simulink model "my_system_ml"  (R2023a)
settings: Solver=VariableStepAuto  StartTime=0.0  StopTime=0.5  MaxStep=1e-6  RelTol=1e-3
undefined symbols (not defined in the file or in its folder): DiscIntNeverNeededParam, Ts, Ts_motor
libraries: slpidlib x50, nesl_utility x20, ee_lib x10, fl_lib x9, simulink x2, rllib x2, spsPWMGeneratorDCDCLib x1, sdl_lib x1, aerolibatmos2 x1
(part 1 of 2)
settings Model: Creator=evloev.saifuddin  LastModifiedBy=evloev.saifuddin

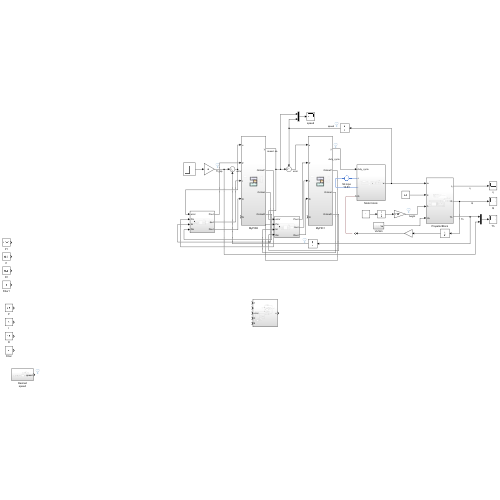
[thumbnail: Simulink's stored preview of the top-level diagram]
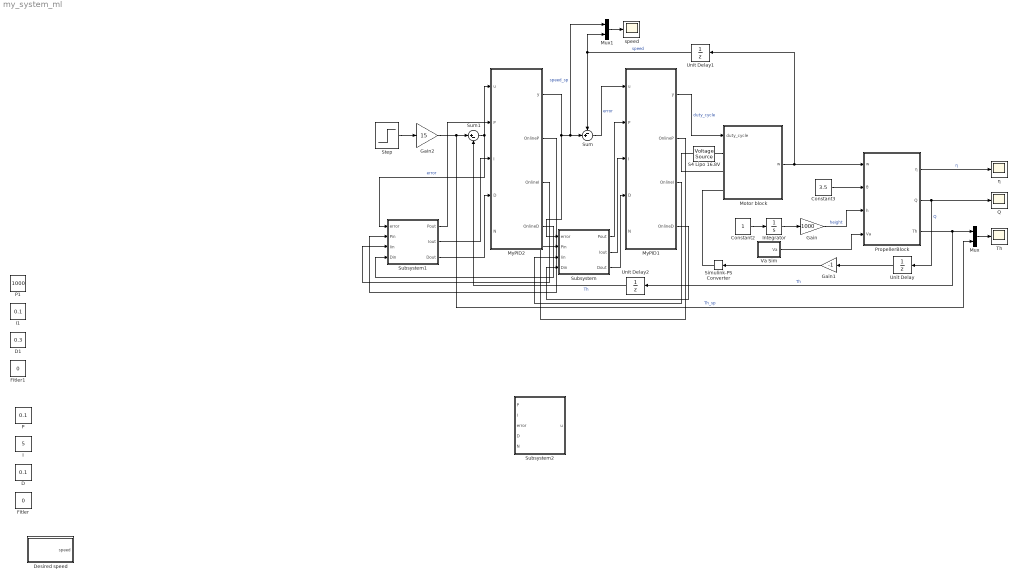
== system my_system_ml ==
  Constant2 : Constant
  Constant3 : Constant  Value=3.5
  D : Constant  Value=0.1
  D1 : Constant  Value=0.3
  Desired speed : Subsystem
  Fitler : Constant  Value=0
  Fitler1 : Constant  Value=0
  Gain : Gain  Gain=1000
  Gain1 : Gain  Gain=-1
  Gain2 : Gain  Gain=15
  I : Constant  Value=5
  I1 : Constant  Value=0.1
  Integrator : Integrator
  Motor block : Subsystem
  Mux : Mux  Inputs=2
  Mux1 : Mux  Inputs=2
  MyPID1 : Subsystem
  MyPID2 : Subsystem
  P : Constant  Value=0.1
  P1 : Constant  Value=1000
  PropellerBlock : Subsystem
  Q : Scope
  S4 Lipo 16.8V : ee_lib/Sources/Voltage Source  dc_voltage=500 V  ac_voltage=0 V  ac_shift=0 rad  ac_frequency=0 Hz  noise_mode=ee.enum.sources.noise.Disabled  PSD=0 V^2/Hz  sample_time=1e-3 s  repeatability=ee.enum.sources.repeatability.NotRepeatable  user_seed=0  auto_seed=19903842  i_specify=off  i_priority=None  i=0 A  i_nominal_specify=off  i_nominal_unit=A  i_nominal_value=1  v_specify=off  v_priority=None  v=0 V  v_nominal_specify=off  v_nominal_unit=V  v_nominal_value=1
  Simulink-PS Converter : nesl_utility/Simulink-PS Converter  PhysicalDomain=network_engine_domain  SubClassName=ps_input  LeftPortType=input  RightPortType=output  PseudoPeriodic=off  Frequencies=[]  NoiseDistribution=none  NoiseParameters=[]  Unit=N*m  AffineConversion=off  FilteringAndDerivatives=provide  SimscapeFilterOrder=1  InputFilterTimeConstant=0.001  UdotUserProvided=0
  Step : Step  Time=0.1  SampleTime=0
  Subsystem : Subsystem
  Subsystem1 : Subsystem
  Subsystem2 : Subsystem
  Sum : Sum  Inputs=-+|
  Sum1 : Sum  Inputs=|+-
  Th : Scope
  Unit Delay : UnitDelay  SampleTime=-1  HasFrameUpgradeWarning=on
  Unit Delay1 : UnitDelay  SampleTime=-1  HasFrameUpgradeWarning=on
  Unit Delay2 : UnitDelay  SampleTime=-1  HasFrameUpgradeWarning=on
  Va Sim : Subsystem
  speed : Scope
  η : Scope
  wires:
  Integrator/1 -> Gain/1
  PropellerBlock/1(η) -> η/1  "η"
  Constant3/1 -> PropellerBlock/2(θ)
  PropellerBlock/3(Th) -> Mux/1, Unit Delay2/1  "Th"
  Gain/1 -> PropellerBlock/3(h)  "height"
  Constant2/1 -> Integrator/1
  Unit Delay/1 -> Gain1/1
  PropellerBlock/2(Q) -> Unit Delay/1, Q/1  "Q"
  Gain1/1 -> Simulink-PS Converter/1
  Unit Delay1/1 -> Mux1/2, Sum/1  "speed"
  Va Sim/1(Va) -> PropellerBlock/4(Va)
  MyPID2/1(y) -> Subsystem/1(error), Mux1/1, Sum/2  "speed_sp"
  Sum1/1 -> MyPID2/1(u), Subsystem1/1(error)  "error"
  Gain2/1 -> Mux/2, Sum1/1  "Th_sp"
  Unit Delay2/1 -> Sum1/2  "Th"
  Motor block/1(w) -> Unit Delay1/1, PropellerBlock/1(w)
  Sum/1 -> MyPID1/1(u)  "error"
  MyPID1/1(y) -> Motor block/1(duty_cycle)  "duty_cycle"
  Mux/1 -> Th/1
  Step/1 -> Gain2/1
  Mux1/1 -> speed/1
  MyPID1/2(OnlineP) -> Subsystem/2(Pin)
  MyPID1/3(OnlineI) -> Subsystem/3(Iin)
  MyPID1/4(OnlineD) -> Subsystem/4(Din)
  Subsystem/1(Pout) -> MyPID1/2(P)
  Subsystem/2(Iout) -> MyPID1/3(I)
  Subsystem/3(Dout) -> MyPID1/4(D)
  Subsystem1/1(Pout) -> MyPID2/2(P)
  Subsystem1/2(Iout) -> MyPID2/3(I)
  Subsystem1/3(Dout) -> MyPID2/4(D)
  MyPID2/4(OnlineD) -> Subsystem1/4(Din)
  MyPID2/3(OnlineI) -> Subsystem1/3(Iin)
  MyPID2/2(OnlineP) -> Subsystem1/2(Pin)
  connections:
  S4 Lipo 16.8V/LConn1 -- Motor block/LConn1
  S4 Lipo 16.8V/RConn1 -- Motor block/LConn2
  Simulink-PS Converter/RConn1 -- Motor block/LConn3

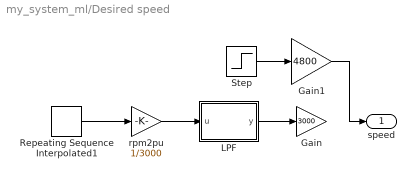
== system my_system_ml/Desired speed ==
  Gain : Gain  Gain=3000
  Gain1 : Gain  Gain=4800
  LPF : Subsystem
  Repeating Sequence Interpolated1 : simulink/Sources/Repeating Sequence Interpolated  OutValues=[0 1025/2 1025/2 1025 1025 2050 2050 2050]  TimeValues=[0 1 2 3 4 5 6 7]/2  LookUpMeth=Interpolation-Use End Values  tsamp=Ts_motor  OutMin=[]  OutMax=[]  OutDataTypeStr=double  OutputDataTypeScalingMode=double  OutDataType=fixdt(0,8)  OutScaling=2^-10
  Step : Step  Time=0.1  SampleTime=0
  rpm2pu : Gain  Gain=1/3000  RndMeth=Simplest  OutDataTypeStr=Inherit: Same as input
  speed : Outport
  wires:
  Repeating Sequence Interpolated1/1 -> rpm2pu/1
  rpm2pu/1 -> LPF/1(u)
  LPF/1(y) -> Gain/1
  Step/1 -> Gain1/1
  Gain1/1 -> speed/1

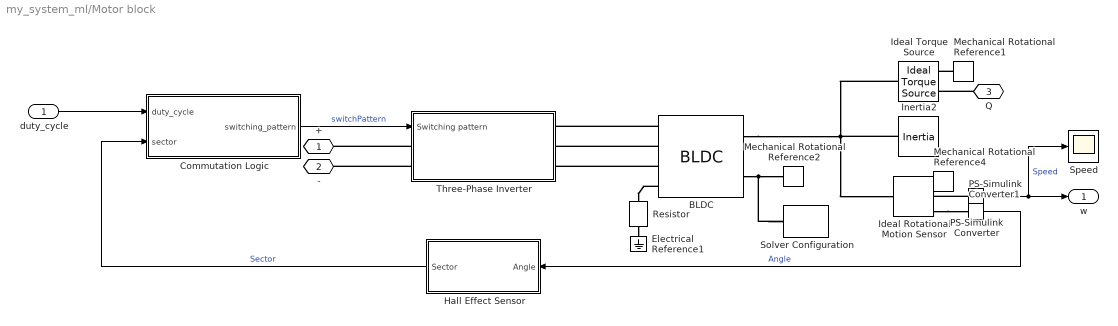
== system my_system_ml/Motor block ==
  duty_cycle : Inport
  BLDC : ee_lib/Electromechanical/Permanent Magnet/BLDC  port_option=ee.enum.threePhasePort.expanded  winding_type=ee.enum.statorconnection.wye  rotor_param=1  pm_flux_linkage=0.00043 Wb  theta_constant=120/7 deg  emf_max=9.6 V  w_meas=600 rpm  DphiDtheta_tab=[0, -.1528, -.1528, .1528, .1528, 0] Wb/rad  back_emf_tab=[0, -9.6, -9.6, 9.6, 9.6, 0] V  rotor_angle_tab=[0, 7.5, 22.5, 37.5, 52.5, 60] deg  nPolePairs=7  axes_param=ee.enum.rotorangle.qaxis  stator_param=ee.enum.statorparam.LdLqL0  machine_param=ee.enum.dqparameterization.constant  Ld=0.000022 H  Lq=0.000022 H  idVec=[-200, 0, 200] A  iqVec=[-200, 0, 200] A  LdMatrix=0.00022 * ones(3, 3) H  LqMatrix=0.00022 * ones(3, 3) H  L0=0.00016 H  Ls=0.0002 H  Lm=0 H  Ms=0.00002 H  Rs=37 mOhm  zero_sequence=ee.enum.park.zerosequence.include  loss_param=ee.enum.ironloss.none  losses_oc=[0, 0, 0] W  losses_sc=[0, 0, 0] W  f_losses=60 Hz  Isc_losses=95 A  J=1.5e-6 kg*m^2  lam=1e-7 N*m/(rad/s)  i_d_specify=off  i_d_priority=None  i_d=0 A  i_d_nominal_specify=off  i_d_nominal_unit=A  i_d_nominal_value=1  i_q_specify=off  i_q_priority=None  i_q=0 A  i_q_nominal_specify=off  i_q_nominal_unit=A  i_q_nominal_value=1  torque_specify=off  torque_priority=None  torque=0 N*m  torque_nominal_specify=off  torque_nominal_unit=N*m  torque_nominal_value=1  angular_velocity_specify=off  angular_velocity_priority=High  angular_velocity=0 rpm  angular_velocity_nominal_specify=off  angular_velocity_nominal_unit=rpm  angular_velocity_nominal_value=1  angular_position_specify=off  angular_position_priority=High  angular_position=0 deg  angular_position_nominal_specify=off  angular_position_nominal_unit=deg  angular_position_nominal_value=1  alpha=3.93e-3 1/K  alpha_flux=-0.001 1/K  Tmeas=298.15 K  stator_thermal_mass=100 J/K  rotor_thermal_mass=200 J/K  Rm_percent_rotor=90  Rd_percent_rotor=30  temperatureA_specify=off  temperatureA_priority=High  temperatureA=25 degC  temperatureA_nominal_specify=off  temperatureA_nominal_unit=degC  temperatureA_nominal_value=1  temperatureB_specify=off  temperatureB_priority=High  temperatureB=25 degC  temperatureB_nominal_specify=off  temperatureB_nominal_unit=degC  temperatureB_nominal_value=1  temperatureC_specify=off  temperatureC_priority=High  temperatureC=25 degC  temperatureC_nominal_specify=off  temperatureC_nominal_unit=degC  temperatureC_nominal_value=1  temperatureR_specify=off  temperatureR_priority=High  temperatureR=25 degC  temperatureR_nominal_specify=off  temperatureR_nominal_unit=degC  temperatureR_nominal_value=1
      settings: InternalSimscapePortConfiguration="{\"Bottom\":[],\"Left\":[{\"id\":\"a\",\"label\":\"a\",\"type\":\"foundation.electrical.electrical\"},{\"id\":\"b\",\"label\":\"b\",\"type\":\"foundation.electrical.electrical\"},{\"id\":\"c\",\"label\":\"c\",\"type\":\"foundation.electrical.electrical\"},{\"id\":\"n\",\"label\":\"n\",\"type\":\"foundation.electrical.electrical\"}],\"Right\":[{\"id\":\"R\",\"label\":\"R\",\"type\":\"foundation.mechanical.rotational.rotational\"},{\"id\":\"C\",\"label\":\"C\",\"type\":\"foundation.mechanical.rotational.rotational\"}],\"Top\":[]}"
  Commutation Logic : Subsystem
  Electrical Reference1 : fl_lib/Electrical/Electrical Elements/Electrical Reference
  Hall Effect Sensor : Subsystem
  Ideal Rotational Motion Sensor : fl_lib/Mechanical/Mechanical Sensors/Ideal Rotational Motion Sensor  reference=foundation.enum.MeasurementReference.difference  acceleration_port=false  velocity_port=true  position_port=true  wrap_angle=false  offset=0 deg
  Ideal Torque Source : fl_lib/Mechanical/Mechanical Sources/Ideal Torque Source
  Inertia2 : fl_lib/Mechanical/Rotational Elements/Inertia  inertia=5.4e-6 kg*m^2  num_ports=foundation.enum.numPorts2.one  w_specify=off  w_priority=High  w=0 rad/s  w_nominal_specify=off  w_nominal_unit=rad/s  w_nominal_value=1  t_specify=off  t_priority=None  t=0 N*m  t_nominal_specify=off  t_nominal_unit=N*m  t_nominal_value=1
  Mechanical Rotational Reference1 : fl_lib/Mechanical/Rotational Elements/Mechanical Rotational Reference
  Mechanical Rotational Reference2 : fl_lib/Mechanical/Rotational Elements/Mechanical Rotational Reference
  Mechanical Rotational Reference4 : fl_lib/Mechanical/Rotational Elements/Mechanical Rotational Reference
  PS-Simulink Converter : nesl_utility/PS-Simulink Converter  PhysicalDomain=network_engine_domain  SubClassName=ps_output  LeftPortType=input  RightPortType=output  PseudoPeriodic=off  Frequencies=[]  VectorFormat=1-D array  Unit=rad/s  AffineConversion=off
  PS-Simulink Converter1 : nesl_utility/PS-Simulink Converter  PhysicalDomain=network_engine_domain  SubClassName=ps_output  LeftPortType=input  RightPortType=output  PseudoPeriodic=off  Frequencies=[]  VectorFormat=1-D array  Unit=deg  AffineConversion=off
  Resistor : fl_lib/Electrical/Electrical Elements/Resistor  R=1e9 Ohm  i_specify=off  i_priority=None  i=0 A  i_nominal_specify=off  i_nominal_unit=A  i_nominal_value=1  v_specify=off  v_priority=None  v=0 V  v_nominal_specify=off  v_nominal_unit=V  v_nominal_value=1
  Solver Configuration : nesl_utility/Solver Configuration  PhysicalDomain=network_engine_domain  SubClassName=solver  LeftPortType=input  RightPortType=generic  Tones=[]  Harmonics=[]  SimulateNoise=off  Profile=off  UseLocalSampling=off  EnableSwitchedLinearOptims=on  FrequencyDomain=off  UseCCode=off  RelTol=0.001  AbsTol=1e-06  MinStep=1e-09  ToWorkspace=off  RevertToSquareIcSolve=off  NumHomotopyIterations=100  PhasorMode=off  PhasorModeNumHarmonics=1  ConsistencySolver=NEWTON_FTOL  IndexReductionMethod=DerivativeReplacement  DoDC=off  ResidualTolerance=1e-09  ConsistencyTolSource=GLOBAL  ConsistencyAbsTol=0.001  ConsistencyRelTol=0.001  ConsistencyTolFactor=0.001  UseLocalSolver=on  LocalSolverChoice=NE_BACKWARD_EULER_ADVANCER  ResolveIndetEquations=on  FunctionEvalNumThread=1  LocalSolverSampleTime=1e-6  DoFixedCost=on  MaxNonlinIter=4  MaxModeIter=2  ComputeImpulses=off  ImpulseIterations=2  LinearAlgebra=auto  LinearAlgebraNumThread=0  EquationFormulation=NE_TIME_EF  DelaysMemoryBudget=1024  AutomaticFiltering=off  FilteringTimeConstant=0.001  PartitionStorageMethod=AS_NEEDED  PartitionMemoryBudget=1024  PartitionMethod=ROBUST
  Speed : Scope
  Three-Phase Inverter : Subsystem
  + : PMIOPort  Side=Left
  - : PMIOPort  Port=2  Side=Left
  Q : PMIOPort  Port=3  Side=Left
  w : Outport
  wires:
  Commutation Logic/1("  switching_pattern") -> Three-Phase Inverter/1(Switching pattern)  "switchPattern"
  PS-Simulink Converter/1 -> Speed/1, w/1  "Speed"
  PS-Simulink Converter1/1 -> Hall Effect Sensor/1(Angle)  "Angle"
  Hall Effect Sensor/1(Sector) -> Commutation Logic/2(sector)  "Sector"
  duty_cycle/1 -> Commutation Logic/1(duty_cycle)
  connections:
  BLDC/RConn1 -- Ideal Torque Source/LConn1 -- Inertia2/LConn1 -- Ideal Rotational Motion Sensor/LConn1
  Three-Phase Inverter/LConn2 -- -/RConn1
  BLDC/LConn1 -- Three-Phase Inverter/RConn1
  PS-Simulink Converter/LConn1 -- Ideal Rotational Motion Sensor/RConn2
  Mechanical Rotational Reference4/LConn1 -- Ideal Rotational Motion Sensor/RConn1
  BLDC/LConn2 -- Three-Phase Inverter/RConn2
  BLDC/LConn4 -- Resistor/LConn1
  BLDC/RConn2 -- Solver Configuration/RConn1 -- Mechanical Rotational Reference2/LConn1
  Ideal Rotational Motion Sensor/RConn3 -- PS-Simulink Converter1/LConn1
  BLDC/LConn3 -- Three-Phase Inverter/RConn3
  Three-Phase Inverter/LConn1 -- +/RConn1
  Mechanical Rotational Reference1/LConn1 -- Ideal Torque Source/RConn2
  Q/RConn1 -- Ideal Torque Source/RConn1
  Resistor/RConn1 -- Electrical Reference1/LConn1

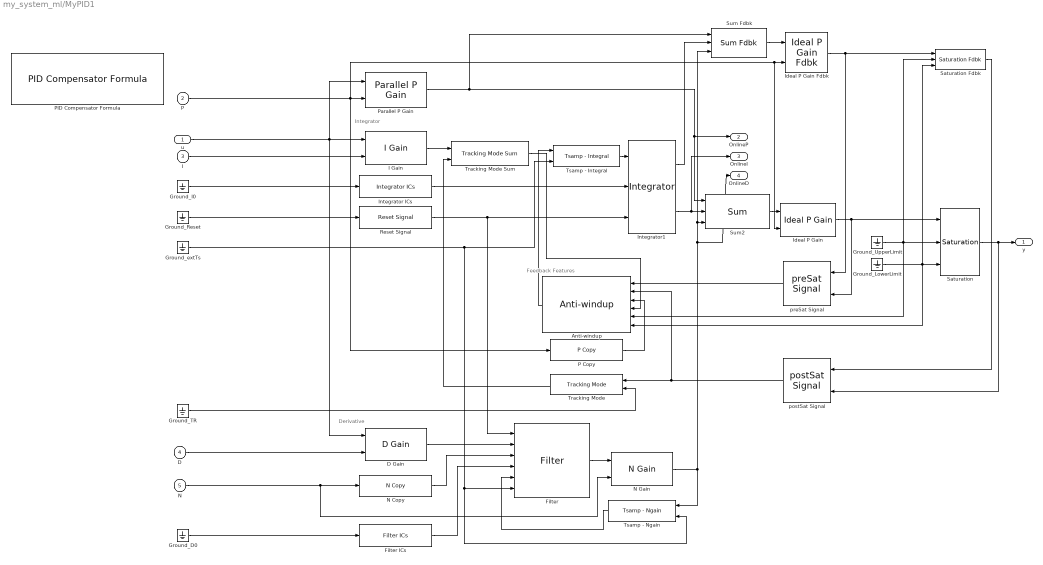
== system my_system_ml/MyPID1 ==
  note: Derivative
  note: Feedback Features
  note: Integrator
  u : Inport
  P : Inport  Port=2
  I : Inport  Port=3
  D : Inport  Port=4
  N : Inport  Port=5
  Anti-windup : slpidlib/PID Controller/Anti-windup  SystemSampleTime=-1  VariantControl=Variant1  LabelModeActiveChoice=BackCalculation  VariantActivationTime=update diagram  Latency=0  AutoFrameSizeCalculation=off
  D Gain : slpidlib/PID Controller/D Gain  SystemSampleTime=-1  VariantControl=Variant1  LabelModeActiveChoice=ExternalParameters  VariantActivationTime=update diagram  Latency=0  AutoFrameSizeCalculation=off
  Filter : slpidlib/PID Controller/Filter  SystemSampleTime=-1  LabelModeActiveChoice=ForwardEulerFilter  VariantActivationTime=update diagram  Latency=0  AutoFrameSizeCalculation=off
  Filter ICs : slpidlib/PID Controller/Filter ICs  SystemSampleTime=-1  VariantControl=Variant1  LabelModeActiveChoice=InternalICsFilter  VariantActivationTime=update diagram  Latency=0  AutoFrameSizeCalculation=off
  Ground_D0 : Ground
  Ground_I0 : Ground
  Ground_LowerLimit : Ground
  Ground_Reset : Ground  DisableCoverage=on
  Ground_TR : Ground  DisableCoverage=on
  Ground_UpperLimit : Ground
  Ground_extTs : Ground
  I Gain : slpidlib/PID Controller/I Gain  SystemSampleTime=-1  VariantControl=Variant1  LabelModeActiveChoice=ExternalParameters  VariantActivationTime=update diagram  Latency=0  AutoFrameSizeCalculation=off
  Ideal P Gain : slpidlib/PID Controller/Ideal P Gain  SystemSampleTime=-1  VariantControl=Variant1  LabelModeActiveChoice=Disabled  VariantActivationTime=update diagram  Latency=0  AutoFrameSizeCalculation=off
  Ideal P Gain Fdbk : slpidlib/PID Controller/Ideal P Gain Fdbk  SystemSampleTime=-1  VariantControl=Variant1  LabelModeActiveChoice=Disabled  VariantActivationTime=update diagram  Latency=0  AutoFrameSizeCalculation=off
  Integrator ICs : slpidlib/PID Controller/Integrator ICs  SystemSampleTime=-1  VariantControl=Variant1  LabelModeActiveChoice=InternalICs  VariantActivationTime=update diagram  Latency=0  AutoFrameSizeCalculation=off
  Integrator1 : slpidlib/PID Controller/Integrator  SystemSampleTime=-1  LabelModeActiveChoice=Discrete  VariantActivationTime=update diagram  Latency=0  AutoFrameSizeCalculation=off
  N Copy : slpidlib/PID Controller/N Copy  SystemSampleTime=-1  LabelModeActiveChoice=Disabled  VariantActivationTime=update diagram  Latency=0  AutoFrameSizeCalculation=off
  N Gain : slpidlib/PID Controller/N Gain  SystemSampleTime=-1  VariantControl=Variant1  LabelModeActiveChoice=ExternalParameters  VariantActivationTime=update diagram  Latency=0  AutoFrameSizeCalculation=off
  P Copy : slpidlib/PID Controller/P Copy  SystemSampleTime=-1  LabelModeActiveChoice=Disabled  VariantActivationTime=update diagram  Latency=0  AutoFrameSizeCalculation=off
  PID Compensator Formula : slpidlib/PID Controller/PID Compensator Formula  SystemSampleTime=-1  VariantActivationTime=update diagram  Latency=0  AutoFrameSizeCalculation=off
  Parallel P Gain : slpidlib/PID Controller/Parallel P Gain  SystemSampleTime=-1  VariantControl=Variant1  LabelModeActiveChoice=ExternalParameters  VariantActivationTime=update diagram  Latency=0  AutoFrameSizeCalculation=off
  Reset Signal : slpidlib/PID Controller/Reset Signal  SystemSampleTime=-1  VariantControl=Variant1  LabelModeActiveChoice=Disabled  VariantActivationTime=update diagram  Latency=0  AutoFrameSizeCalculation=off
  Saturation : slpidlib/PID Controller/Saturation  SystemSampleTime=-1  LabelModeActiveChoice=Enabled  VariantActivationTime=update diagram  Latency=0  AutoFrameSizeCalculation=off
  Saturation Fdbk : slpidlib/PID Controller/Saturation Fdbk  SystemSampleTime=-1  LabelModeActiveChoice=Disabled  VariantActivationTime=update diagram  Latency=0  AutoFrameSizeCalculation=off
  Sum Fdbk : slpidlib/PID Controller/Sum Fdbk  DisableCoverage=on  SystemSampleTime=-1  LabelModeActiveChoice=Disabled  VariantActivationTime=update diagram  Latency=0  AutoFrameSizeCalculation=off
  Sum2 : slpidlib/PID Controller/Sum  SystemSampleTime=-1  LabelModeActiveChoice=Sum_PID  VariantActivationTime=update diagram  Latency=0  AutoFrameSizeCalculation=off
  Tracking Mode : slpidlib/PID Controller/Tracking Mode  SystemSampleTime=-1  VariantControl=Variant1  LabelModeActiveChoice=Disabled  VariantActivationTime=update diagram  Latency=0  AutoFrameSizeCalculation=off
  Tracking Mode Sum : slpidlib/PID Controller/Tracking Mode Sum  SystemSampleTime=-1  LabelModeActiveChoice=Passthrough  VariantActivationTime=update diagram  Latency=0  AutoFrameSizeCalculation=off
  Tsamp - Integral : slpidlib/PID Controller/Tsamp - Integral  SystemSampleTime=-1  LabelModeActiveChoice=Disabled_SignalSpec  VariantActivationTime=update diagram  Latency=0  AutoFrameSizeCalculation=off
  Tsamp - Ngain : slpidlib/PID Controller/Tsamp - Ngain  SystemSampleTime=-1  LabelModeActiveChoice=Passthrough  VariantActivationTime=update diagram  Latency=0  AutoFrameSizeCalculation=off
  postSat Signal : slpidlib/PID Controller/postSat Signal  SystemSampleTime=-1  VariantControl=Variant1  LabelModeActiveChoice=Forward  VariantActivationTime=update diagram  Latency=0  AutoFrameSizeCalculation=off
  preSat Signal : slpidlib/PID Controller/preSat Signal  SystemSampleTime=-1  VariantControl=Variant1  LabelModeActiveChoice=Forward  VariantActivationTime=update diagram  Latency=0  AutoFrameSizeCalculation=off
  y : Outport
  OnlineP : Outport  Port=2
  OnlineI : Outport  Port=3
  OnlineD : Outport  Port=4
  wires:
  Ground_Reset/1 -> Reset Signal/1
  Tsamp - Ngain/1 -> Filter/5
  Ideal P Gain Fdbk/1 -> preSat Signal/1, Saturation Fdbk/1
  Saturation/1 -> y/1, postSat Signal/2
  Ground_extTs/1 -> Tsamp - Integral/2, Filter/6, Tsamp - Ngain/2
  Filter/1 -> N Gain/1
  I/1 -> I Gain/2
  Filter ICs/1 -> Filter/4
  Tracking Mode/1 -> Tracking Mode Sum/2
  N/1 -> N Copy/1, N Gain/2
  Ground_I0/1 -> Integrator ICs/1
  Tsamp - Integral/1 -> Integrator1/1
  Parallel P Gain/1 -> Sum2/1, OnlineP/1, Sum Fdbk/1
  Reset Signal/1 -> Filter/1, Integrator1/3
  Ground_D0/1 -> Filter ICs/1
  Ground_LowerLimit/1 -> Saturation/3, Anti-windup/6, Saturation Fdbk/3
  P Copy/1 -> Anti-windup/3
  Integrator1/1 -> Sum Fdbk/2
  Anti-windup/1 -> Tsamp - Integral/1
  Ideal P Gain/1 -> Saturation/1, preSat Signal/2
  Integrator1/2 -> Sum2/2, OnlineI/1
  Ground_UpperLimit/1 -> Saturation/2, Saturation Fdbk/2, Anti-windup/5
  u/1 -> D Gain/1, I Gain/1, Parallel P Gain/1
  Sum Fdbk/1 -> Ideal P Gain Fdbk/1
  preSat Signal/1 -> Anti-windup/1
  P/1 -> Ideal P Gain Fdbk/2, Ideal P Gain/2, Parallel P Gain/2, P Copy/1
  D Gain/1 -> Filter/2
  Saturation Fdbk/1 -> postSat Signal/1
  Integrator ICs/1 -> Integrator1/2
  Sum2/1 -> Ideal P Gain/1
  N Copy/1 -> Filter/3
  Ground_TR/1 -> Tracking Mode/2
  Tracking Mode Sum/1 -> Anti-windup/4
  postSat Signal/1 -> Tracking Mode/1, Anti-windup/2
  I Gain/1 -> Tracking Mode Sum/1
  D/1 -> D Gain/2
  N Gain/1 -> Tsamp - Ngain/1, Sum Fdbk/3, Sum2/3, OnlineD/1

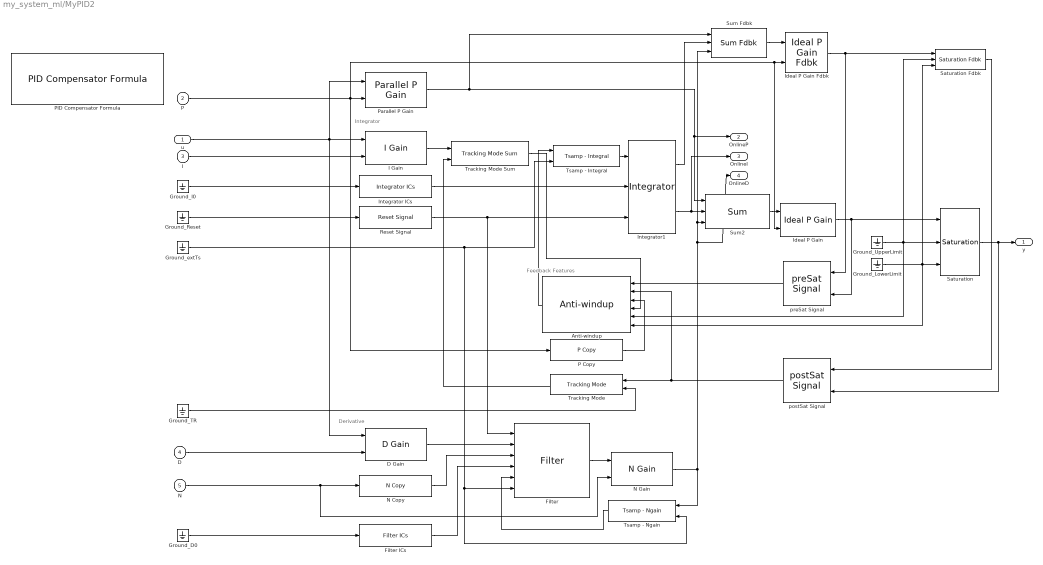
== system my_system_ml/MyPID2 ==
  note: Derivative
  note: Feedback Features
  note: Integrator
  u : Inport
  P : Inport  Port=2
  I : Inport  Port=3
  D : Inport  Port=4
  N : Inport  Port=5
  Anti-windup : slpidlib/PID Controller/Anti-windup  SystemSampleTime=-1  VariantControl=Variant1  LabelModeActiveChoice=BackCalculation  VariantActivationTime=update diagram  Latency=0  AutoFrameSizeCalculation=off
  D Gain : slpidlib/PID Controller/D Gain  SystemSampleTime=-1  VariantControl=Variant1  LabelModeActiveChoice=ExternalParameters  VariantActivationTime=update diagram  Latency=0  AutoFrameSizeCalculation=off
  Filter : slpidlib/PID Controller/Filter  SystemSampleTime=-1  LabelModeActiveChoice=ForwardEulerFilter  VariantActivationTime=update diagram  Latency=0  AutoFrameSizeCalculation=off
  Filter ICs : slpidlib/PID Controller/Filter ICs  SystemSampleTime=-1  VariantControl=Variant1  LabelModeActiveChoice=InternalICsFilter  VariantActivationTime=update diagram  Latency=0  AutoFrameSizeCalculation=off
  Ground_D0 : Ground
  Ground_I0 : Ground
  Ground_LowerLimit : Ground
  Ground_Reset : Ground  DisableCoverage=on
  Ground_TR : Ground  DisableCoverage=on
  Ground_UpperLimit : Ground
  Ground_extTs : Ground
  I Gain : slpidlib/PID Controller/I Gain  SystemSampleTime=-1  VariantControl=Variant1  LabelModeActiveChoice=ExternalParameters  VariantActivationTime=update diagram  Latency=0  AutoFrameSizeCalculation=off
  Ideal P Gain : slpidlib/PID Controller/Ideal P Gain  SystemSampleTime=-1  VariantControl=Variant1  LabelModeActiveChoice=Disabled  VariantActivationTime=update diagram  Latency=0  AutoFrameSizeCalculation=off
  Ideal P Gain Fdbk : slpidlib/PID Controller/Ideal P Gain Fdbk  SystemSampleTime=-1  VariantControl=Variant1  LabelModeActiveChoice=Disabled  VariantActivationTime=update diagram  Latency=0  AutoFrameSizeCalculation=off
  Integrator ICs : slpidlib/PID Controller/Integrator ICs  SystemSampleTime=-1  VariantControl=Variant1  LabelModeActiveChoice=InternalICs  VariantActivationTime=update diagram  Latency=0  AutoFrameSizeCalculation=off
  Integrator1 : slpidlib/PID Controller/Integrator  SystemSampleTime=-1  LabelModeActiveChoice=Discrete  VariantActivationTime=update diagram  Latency=0  AutoFrameSizeCalculation=off
  N Copy : slpidlib/PID Controller/N Copy  SystemSampleTime=-1  LabelModeActiveChoice=Disabled  VariantActivationTime=update diagram  Latency=0  AutoFrameSizeCalculation=off
  N Gain : slpidlib/PID Controller/N Gain  SystemSampleTime=-1  VariantControl=Variant1  LabelModeActiveChoice=ExternalParameters  VariantActivationTime=update diagram  Latency=0  AutoFrameSizeCalculation=off
  P Copy : slpidlib/PID Controller/P Copy  SystemSampleTime=-1  LabelModeActiveChoice=Disabled  VariantActivationTime=update diagram  Latency=0  AutoFrameSizeCalculation=off
  PID Compensator Formula : slpidlib/PID Controller/PID Compensator Formula  SystemSampleTime=-1  VariantActivationTime=update diagram  Latency=0  AutoFrameSizeCalculation=off
  Parallel P Gain : slpidlib/PID Controller/Parallel P Gain  SystemSampleTime=-1  VariantControl=Variant1  LabelModeActiveChoice=ExternalParameters  VariantActivationTime=update diagram  Latency=0  AutoFrameSizeCalculation=off
  Reset Signal : slpidlib/PID Controller/Reset Signal  SystemSampleTime=-1  VariantControl=Variant1  LabelModeActiveChoice=Disabled  VariantActivationTime=update diagram  Latency=0  AutoFrameSizeCalculation=off
  Saturation : slpidlib/PID Controller/Saturation  SystemSampleTime=-1  LabelModeActiveChoice=Enabled  VariantActivationTime=update diagram  Latency=0  AutoFrameSizeCalculation=off
  Saturation Fdbk : slpidlib/PID Controller/Saturation Fdbk  SystemSampleTime=-1  LabelModeActiveChoice=Disabled  VariantActivationTime=update diagram  Latency=0  AutoFrameSizeCalculation=off
  Sum Fdbk : slpidlib/PID Controller/Sum Fdbk  DisableCoverage=on  SystemSampleTime=-1  LabelModeActiveChoice=Disabled  VariantActivationTime=update diagram  Latency=0  AutoFrameSizeCalculation=off
  Sum2 : slpidlib/PID Controller/Sum  SystemSampleTime=-1  LabelModeActiveChoice=Sum_PID  VariantActivationTime=update diagram  Latency=0  AutoFrameSizeCalculation=off
  Tracking Mode : slpidlib/PID Controller/Tracking Mode  SystemSampleTime=-1  VariantControl=Variant1  LabelModeActiveChoice=Disabled  VariantActivationTime=update diagram  Latency=0  AutoFrameSizeCalculation=off
  Tracking Mode Sum : slpidlib/PID Controller/Tracking Mode Sum  SystemSampleTime=-1  LabelModeActiveChoice=Passthrough  VariantActivationTime=update diagram  Latency=0  AutoFrameSizeCalculation=off
  Tsamp - Integral : slpidlib/PID Controller/Tsamp - Integral  SystemSampleTime=-1  LabelModeActiveChoice=Disabled_SignalSpec  VariantActivationTime=update diagram  Latency=0  AutoFrameSizeCalculation=off
  Tsamp - Ngain : slpidlib/PID Controller/Tsamp - Ngain  SystemSampleTime=-1  LabelModeActiveChoice=Passthrough  VariantActivationTime=update diagram  Latency=0  AutoFrameSizeCalculation=off
  postSat Signal : slpidlib/PID Controller/postSat Signal  SystemSampleTime=-1  VariantControl=Variant1  LabelModeActiveChoice=Forward  VariantActivationTime=update diagram  Latency=0  AutoFrameSizeCalculation=off
  preSat Signal : slpidlib/PID Controller/preSat Signal  SystemSampleTime=-1  VariantControl=Variant1  LabelModeActiveChoice=Forward  VariantActivationTime=update diagram  Latency=0  AutoFrameSizeCalculation=off
  y : Outport
  OnlineP : Outport  Port=2
  OnlineI : Outport  Port=3
  OnlineD : Outport  Port=4
  wires:
  Ground_Reset/1 -> Reset Signal/1
  Tsamp - Ngain/1 -> Filter/5
  Ideal P Gain Fdbk/1 -> preSat Signal/1, Saturation Fdbk/1
  Saturation/1 -> y/1, postSat Signal/2
  Ground_extTs/1 -> Tsamp - Integral/2, Filter/6, Tsamp - Ngain/2
  Filter/1 -> N Gain/1
  I/1 -> I Gain/2
  Filter ICs/1 -> Filter/4
  Tracking Mode/1 -> Tracking Mode Sum/2
  N/1 -> N Copy/1, N Gain/2
  Ground_I0/1 -> Integrator ICs/1
  Tsamp - Integral/1 -> Integrator1/1
  Parallel P Gain/1 -> Sum2/1, OnlineP/1, Sum Fdbk/1
  Reset Signal/1 -> Filter/1, Integrator1/3
  Ground_D0/1 -> Filter ICs/1
  Ground_LowerLimit/1 -> Saturation/3, Anti-windup/6, Saturation Fdbk/3
  P Copy/1 -> Anti-windup/3
  Integrator1/1 -> Sum Fdbk/2
  Anti-windup/1 -> Tsamp - Integral/1
  Ideal P Gain/1 -> Saturation/1, preSat Signal/2
  Integrator1/2 -> Sum2/2, OnlineI/1
  Ground_UpperLimit/1 -> Saturation/2, Saturation Fdbk/2, Anti-windup/5
  u/1 -> D Gain/1, I Gain/1, Parallel P Gain/1
  Sum Fdbk/1 -> Ideal P Gain Fdbk/1
  preSat Signal/1 -> Anti-windup/1
  P/1 -> Ideal P Gain Fdbk/2, Ideal P Gain/2, Parallel P Gain/2, P Copy/1
  D Gain/1 -> Filter/2
  Saturation Fdbk/1 -> postSat Signal/1
  Integrator ICs/1 -> Integrator1/2
  Sum2/1 -> Ideal P Gain/1
  N Copy/1 -> Filter/3
  Ground_TR/1 -> Tracking Mode/2
  Tracking Mode Sum/1 -> Anti-windup/4
  postSat Signal/1 -> Tracking Mode/1, Anti-windup/2
  I Gain/1 -> Tracking Mode Sum/1
  D/1 -> D Gain/2
  N Gain/1 -> Tsamp - Ngain/1, Sum Fdbk/3, Sum2/3, OnlineD/1

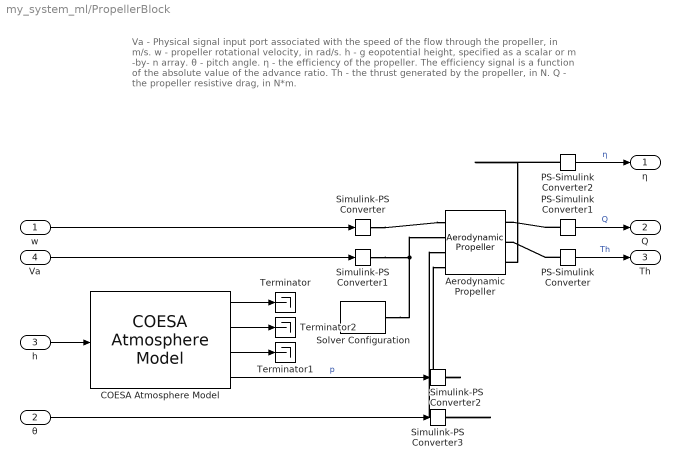
== system my_system_ml/PropellerBlock ==
  note: Va - Physical signal input port associated with the speed of the flow through the propeller, in m/s.
      | w - propeller rotational velocity, in rad/s.
      | h - g eopotential height, specified as a scalar or m -by- n array.
      | θ - pitch angle.
      | η - the efficiency of the propeller. The efficiency signal is a function of the absolute value of the advance ratio.
      | Th - the thrust generated by the propeller, in N.
      | Q - the propeller resistive drag, in N*m.
  w : Inport
  θ : Inport  Port=2
  h : Inport  Port=3
  Va : Inport  Port=4
  Aerodynamic Propeller : sdl_lib/Engines & Motors/Aerodynamic Propeller  parameterization=sdl.enum.PropellerParameterization.TabulatedBeta  pitch_type=foundation.enum.constant_controlled.controlled  direction=sdl.enum.PropellerDirection.Positive  D=129.54 mm  kt_const=0.15  kp_const=0.13  kt_poly_fixed=[.002, .0006, -.0509, .0617]  kp_poly_fixed=[-.0752, .0577, -.0622, .16]  pitch_angle_TLU=[22, 23] deg  kt_poly_TLU=[.0002, -.00041, -.036, .03; .00026, -.00056, -.048, .04; .002, .00063, -.051, .062; .0014, -.0016, -.048, .087; .00087, -.0036, -.041, .12]  kp_poly_TLU=[-.1, .031, .0055, .088; -.081, -.025, .0044, .07; -.075, .058, -.062, .16; -.052, .065, -.08, .3; -.031, .057, -.069, .4]  J_TLU=[.01, .3, .625, 1.55, 2, 2.6]  kt_TLU_1D=[.0614, .0473, .0318, -.0127, -.0343, -.063]  kp_TLU_1D=[.1496, .1314, .116, -.0521, -.1503, -.2813]  kt_TLU_2D=[.00019, .013, .0048, -.017, -.03, -.045; .00039, .025, .0096, -.037, -.06, -.09; .00061, .047, .032, -.013, -.034, -.063; .00086, .072, .057, .014, -.0076, -.036; .12, .104, .09, .049, .029, .0019]  kp_TLU_2D=[.029, .029, .016, .06, .009, -.16; .059, .054, .031, -.12, -.19, -.29; .15, .13, .12, -.052, -.15, -.28; .26, .24, .22, .097, -.04, -.25; .39, .39, .38, .32, .24, .062]  beta_TLU=[4.1, 5.1, 6.0, 7.1, 8.0, 9.3, 10.2, 11.3, 12.0, 13.1, 14.3, 15.3, 16.3] deg  Ct_TLU_1D=0.035 * sind(linspace(0, 360, 10) - 200)  Cq_TLU_1D=0.010 * sind(linspace(0, 360, 10) - 200)  Ct_TLU_2D=[[0.0588 0.0554 0.0523 0.0482 0.0437 0.0383 0.0347 0.0296 0.0268 0.0213 0.0146 0.0083 0.0016]; [0.0588 0.0554 0.0523 0.0482 0.0437 0.0383 0.0347 0.0296 0.0268 0.0213 0.0146 0.0083 0.0016]]  Cq_TLU_2D=[[0.00637 0.00629 0.00621 0.00608 0.00586 0.00560 0.00538 0.00505 0.00485 0.00442 0.00388 0.00334 0.00275]; [0.00637 0.00629 0.00621 0.00608 0.00586 0.00560 0.00538 0.00505 0.00485 0.00442 0.00388 0.00334 0.00275]]  interp_method=simscape.enum.interpolation.linear  extrap_method=simscape.enum.extrapolation.linear  density_spec=foundation.enum.constant_variable.variable  rho=1.225 kg/m^3  rotational_ports=sdl.enum.ConnectionType.PS  translational_ports=sdl.enum.ConnectionType.PS  model_inertia=true  propeller_inertia=1 kg*m^2  propeller_mass=10 kg  efficiency_sensor=true  n_thr=0.001 Hz  k_thr=0.001  operation_check=simscape.enum.assert.action.warn  expose_port_C=false  w_specify=off  w_priority=None  w=0 rad/s  w_nominal_specify=off  w_nominal_unit=rad/s  w_nominal_value=1  Q_specify=off  Q_priority=None  Q=0 N*m  Q_nominal_specify=off  Q_nominal_unit=N*m  Q_nominal_value=1  v_specify=off  v_priority=None  v=0 m/s  v_nominal_specify=off  v_nominal_unit=m/s  v_nominal_value=1  thrust_specify=off  thrust_priority=None  thrust=0 N  thrust_nominal_specify=off  thrust_nominal_unit=N  thrust_nominal_value=1
      settings: InternalSimscapePortConfiguration="{\"Bottom\":[{\"id\":\"pitch_in\",\"label\":\"θ\",\"type\":\"input\"},{\"id\":\"rho_in\",\"label\":\"Rho\",\"type\":\"input\"}],\"Left\":[{\"id\":\"Q_out\",\"label\":\"Q\",\"type\":\"output\"},{\"id\":\"Th_out\",\"label\":\"Th\",\"type\":\"output\"}],\"Right\":[{\"id\":\"w_in\",\"label\":\"w\",\"type\":\"input\"},{\"id\":\"Va_in\",\"label\":\"Va\",\"type\":\"input\"}],\"Top\":[{\"id\":\"Eff_out\",\"label\":\"E\",\"type\":\"output\"}]}"
  COESA Atmosphere Model : aerolibatmos2/COESA Atmosphere Model  units=Metric (MKS)  spec=1976 COESA-extended U.S. Standard Atmosphere  model=Profile  profile_var=High temperature  profile_percent=1%  profile_alt=5 km (16404 ft)  envelope_var=High temperature  envelope_percent=1%  action=Warning
  PS-Simulink Converter : nesl_utility/PS-Simulink Converter  PhysicalDomain=network_engine_domain  SubClassName=ps_output  LeftPortType=input  RightPortType=output  PseudoPeriodic=off  Frequencies=[]  VectorFormat=inherit  Unit=N  AffineConversion=off
  PS-Simulink Converter1 : nesl_utility/PS-Simulink Converter  PhysicalDomain=network_engine_domain  SubClassName=ps_output  LeftPortType=input  RightPortType=output  PseudoPeriodic=off  Frequencies=[]  VectorFormat=inherit  Unit=N*m  AffineConversion=off
  PS-Simulink Converter2 : nesl_utility/PS-Simulink Converter  PhysicalDomain=network_engine_domain  SubClassName=ps_output  LeftPortType=input  RightPortType=output  PseudoPeriodic=off  Frequencies=[]  VectorFormat=inherit  Unit=inherit  AffineConversion=off
  Simulink-PS Converter : nesl_utility/Simulink-PS Converter  PhysicalDomain=network_engine_domain  SubClassName=ps_input  LeftPortType=input  RightPortType=output  PseudoPeriodic=off  Frequencies=[]  NoiseDistribution=none  NoiseParameters=[]  Unit=rad/s  AffineConversion=off  FilteringAndDerivatives=provide  SimscapeFilterOrder=1  InputFilterTimeConstant=0.001  UdotUserProvided=0
  Simulink-PS Converter1 : nesl_utility/Simulink-PS Converter  PhysicalDomain=network_engine_domain  SubClassName=ps_input  LeftPortType=input  RightPortType=output  PseudoPeriodic=off  Frequencies=[]  NoiseDistribution=none  NoiseParameters=[]  Unit=m/s  AffineConversion=off  FilteringAndDerivatives=provide  SimscapeFilterOrder=1  InputFilterTimeConstant=0.001  UdotUserProvided=0
  Simulink-PS Converter2 : nesl_utility/Simulink-PS Converter  PhysicalDomain=network_engine_domain  SubClassName=ps_input  LeftPortType=input  RightPortType=output  PseudoPeriodic=off  Frequencies=[]  NoiseDistribution=none  NoiseParameters=[]  Unit=kg/m^3  AffineConversion=off  FilteringAndDerivatives=provide  SimscapeFilterOrder=1  InputFilterTimeConstant=0.001  UdotUserProvided=0
  Simulink-PS Converter3 : nesl_utility/Simulink-PS Converter  PhysicalDomain=network_engine_domain  SubClassName=ps_input  LeftPortType=input  RightPortType=output  PseudoPeriodic=off  Frequencies=[]  NoiseDistribution=none  NoiseParameters=[]  Unit=1  AffineConversion=off  FilteringAndDerivatives=provide  SimscapeFilterOrder=1  InputFilterTimeConstant=0.001  UdotUserProvided=0
  Solver Configuration : nesl_utility/Solver Configuration  PhysicalDomain=network_engine_domain  SubClassName=solver  LeftPortType=input  RightPortType=generic  Tones=[]  Harmonics=[]  SimulateNoise=off  Profile=off  UseLocalSampling=off  EnableSwitchedLinearOptims=on  FrequencyDomain=off  UseCCode=off  RelTol=0.001  AbsTol=0.001  MinStep=1e-09  ToWorkspace=off  RevertToSquareIcSolve=off  NumHomotopyIterations=100  PhasorMode=off  PhasorModeNumHarmonics=1  ConsistencySolver=NEWTON_XTOL_AFTER_FTOL  IndexReductionMethod=DerivativeReplacement  DoDC=off  ResidualTolerance=1e-09  ConsistencyTolSource=GLOBAL  ConsistencyAbsTol=0.001  ConsistencyRelTol=0.001  ConsistencyTolFactor=0.001  UseLocalSolver=off  LocalSolverChoice=NE_BACKWARD_EULER_ADVANCER  ResolveIndetEquations=on  FunctionEvalNumThread=1  LocalSolverSampleTime=0.001  DoFixedCost=off  MaxNonlinIter=3  MaxModeIter=2  ComputeImpulses=off  ImpulseIterations=2  LinearAlgebra=auto  LinearAlgebraNumThread=0  EquationFormulation=NE_TIME_EF  DelaysMemoryBudget=1024  AutomaticFiltering=on  FilteringTimeConstant=0.001  PartitionStorageMethod=AS_NEEDED  PartitionMemoryBudget=1024  PartitionMethod=ROBUST
  Terminator : Terminator
  Terminator1 : Terminator
  Terminator2 : Terminator
  η : Outport
  Q : Outport  Port=2
  Th : Outport  Port=3
  wires:
  PS-Simulink Converter/1 -> Th/1  "Th"
  PS-Simulink Converter1/1 -> Q/1  "Q"
  θ/1 -> Simulink-PS Converter3/1
  h/1 -> COESA Atmosphere Model/1
  COESA Atmosphere Model/4 -> Simulink-PS Converter2/1  "p"
  PS-Simulink Converter2/1 -> η/1  "η"
  w/1 -> Simulink-PS Converter/1
  COESA Atmosphere Model/2 -> Terminator2/1
  Va/1 -> Simulink-PS Converter1/1
  COESA Atmosphere Model/1 -> Terminator/1
  COESA Atmosphere Model/3 -> Terminator1/1
  connections:
  Simulink-PS Converter/RConn1 -- Aerodynamic Propeller/RConn1
  PS-Simulink Converter2/LConn1 -- Aerodynamic Propeller/LConn3
  Simulink-PS Converter1/RConn1 -- Solver Configuration/RConn1 -- Aerodynamic Propeller/RConn2
  Simulink-PS Converter2/RConn1 -- Aerodynamic Propeller/RConn4
  PS-Simulink Converter1/LConn1 -- Aerodynamic Propeller/LConn1
  PS-Simulink Converter/LConn1 -- Aerodynamic Propeller/LConn2
  Simulink-PS Converter3/RConn1 -- Aerodynamic Propeller/RConn3

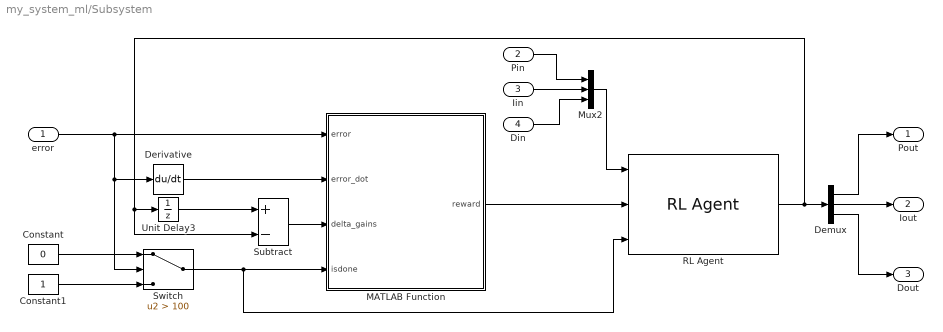
== system my_system_ml/Subsystem ==
  error : Inport
  Pin : Inport  Port=2
  Iin : Inport  Port=3
  Din : Inport  Port=4
  Constant : Constant  Value=0
  Constant1 : Constant
  Demux : Demux  Outputs=3
  Derivative : Derivative
  MATLAB Function : MATLAB Function  TreatAsAtomicUnit=on
  Mux2 : Mux  Inputs=3
  RL Agent : rllib/RL Agent  Agent=agentObj  ExternalActionAsInput=off  ProvideLastAction=off  ProvideCumRwd=off  TreatAsDirectFeedthrough=on  UseStrictObservationDataTypes=off
  Subtract : Sum  Inputs=+-
  Switch : Switch  Criteria=u2 > Threshold  Threshold=100  SaturateOnIntegerOverflow=off  InputSameDT=off
  Unit Delay3 : UnitDelay  SampleTime=-1  HasFrameUpgradeWarning=on
  Pout : Outport
  Iout : Outport  Port=2
  Dout : Outport  Port=3
  wires:
  RL Agent/1 -> Subtract/2, Unit Delay3/1, Demux/1
  Switch/1 -> RL Agent/3, MATLAB Function/4(isdone)
  error/1 -> Derivative/1, Switch/2, MATLAB Function/1(error)
  Pin/1 -> Mux2/1
  Subtract/1 -> MATLAB Function/3(delta_gains)
  Constant1/1 -> Switch/3
  Unit Delay3/1 -> Subtract/1
  Constant/1 -> Switch/1
  MATLAB Function/1(reward) -> RL Agent/2
  Derivative/1 -> MATLAB Function/2(error_dot)
  Mux2/1 -> RL Agent/1
  Iin/1 -> Mux2/2
  Din/1 -> Mux2/3
  Demux/1 -> Pout/1
  Demux/3 -> Dout/1
  Demux/2 -> Iout/1

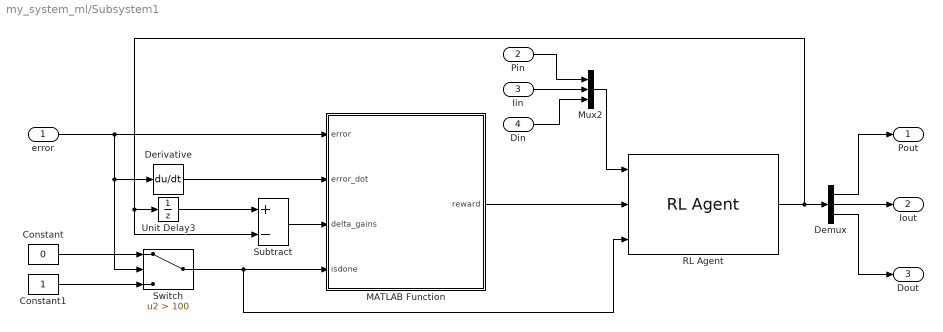
== system my_system_ml/Subsystem1 ==
  error : Inport
  Pin : Inport  Port=2
  Iin : Inport  Port=3
  Din : Inport  Port=4
  Constant : Constant  Value=0
  Constant1 : Constant
  Demux : Demux  Outputs=3
  Derivative : Derivative
  MATLAB Function : MATLAB Function  TreatAsAtomicUnit=on
  Mux2 : Mux  Inputs=3
  RL Agent : rllib/RL Agent  Agent=agentObj  ExternalActionAsInput=off  ProvideLastAction=off  ProvideCumRwd=off  TreatAsDirectFeedthrough=on  UseStrictObservationDataTypes=off
  Subtract : Sum  Inputs=+-
  Switch : Switch  Criteria=u2 > Threshold  Threshold=100  SaturateOnIntegerOverflow=off  InputSameDT=off
  Unit Delay3 : UnitDelay  SampleTime=-1  HasFrameUpgradeWarning=on
  Pout : Outport
  Iout : Outport  Port=2
  Dout : Outport  Port=3
  wires:
  RL Agent/1 -> Subtract/2, Unit Delay3/1, Demux/1
  Switch/1 -> RL Agent/3, MATLAB Function/4(isdone)
  error/1 -> Derivative/1, Switch/2, MATLAB Function/1(error)
  Pin/1 -> Mux2/1
  Subtract/1 -> MATLAB Function/3(delta_gains)
  Constant1/1 -> Switch/3
  Unit Delay3/1 -> Subtract/1
  Constant/1 -> Switch/1
  MATLAB Function/1(reward) -> RL Agent/2
  Derivative/1 -> MATLAB Function/2(error_dot)
  Mux2/1 -> RL Agent/1
  Iin/1 -> Mux2/2
  Din/1 -> Mux2/3
  Demux/1 -> Pout/1
  Demux/3 -> Dout/1
  Demux/2 -> Iout/1

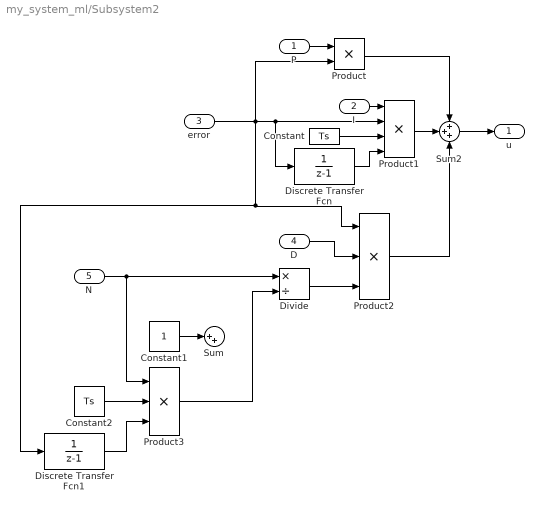
== system my_system_ml/Subsystem2 ==
  P : Inport
  I : Inport  Port=2
  error : Inport  Port=3
  D : Inport  Port=4
  N : Inport  Port=5
  Constant : Constant  Value=Ts
  Constant1 : Constant
  Constant2 : Constant  Value=Ts
  Discrete Transfer Fcn : DiscreteTransferFcn  Denominator=[1 -1]
  Discrete Transfer Fcn1 : DiscreteTransferFcn  Denominator=[1 -1]
  Divide : Product  Inputs=*/
  Product : Product
  Product1 : Product  Inputs=4
  Product2 : Product  Inputs=3
  Product3 : Product  Inputs=3
  Sum : Sum  Inputs=|++
  Sum2 : Sum  Inputs=+++
  u : Outport
  wires:
  error/1 -> Product2/1, Discrete Transfer Fcn1/1, Discrete Transfer Fcn/1, Product1/2, Product/2
  Product2/1 -> Sum2/3
  Sum2/1 -> u/1
  Product1/1 -> Sum2/2
  Constant/1 -> Product1/3
  I/1 -> Product1/1
  P/1 -> Product/1
  Product/1 -> Sum2/1
  Discrete Transfer Fcn/1 -> Product1/4
  Divide/1 -> Product2/3
  N/1 -> Divide/1, Product3/1
  Constant1/1 -> Sum/1
  Constant2/1 -> Product3/2
  Discrete Transfer Fcn1/1 -> Product3/3
  Product3/1 -> Divide/2
  D/1 -> Product2/2

== system my_system_ml/Va Sim ==
  Base Va : Constant  Value=10
  Gain2 : Gain  Gain=10
  Integrator2 : Integrator
  Noise Va : simulink/Sources/Band-Limited White Noise  Cov=[0.5]  Ts=0.1  seed=[23341]
  Sine Wave : Sin  Amplitude=20  Bias=5  SampleTime=0
  Sum1 : Sum  Inputs=+++
  Va : Outport
  wires:
  Noise Va/1 -> Gain2/1
  Base Va/1 -> Sum1/2
  Integrator2/1 -> Sum1/1
  Sine Wave/1 -> Sum1/3
  Gain2/1 -> Integrator2/1
  Sum1/1 -> Va/1  "Va"

== system my_system_ml/Desired speed/LPF ==
  u : Inport
  Discrete-Time Integrator : DiscreteIntegrator  gainval=20  SampleTime=Ts_motor  ICPrevOutput=DiscIntNeverNeededParam  ICPrevScaledInput=DiscIntNeverNeededParam
  Sum : Sum  Inputs=|+-
  y : Outport
  wires:
  Sum/1 -> Discrete-Time Integrator/1
  Discrete-Time Integrator/1 -> y/1, Sum/2
  u/1 -> Sum/1

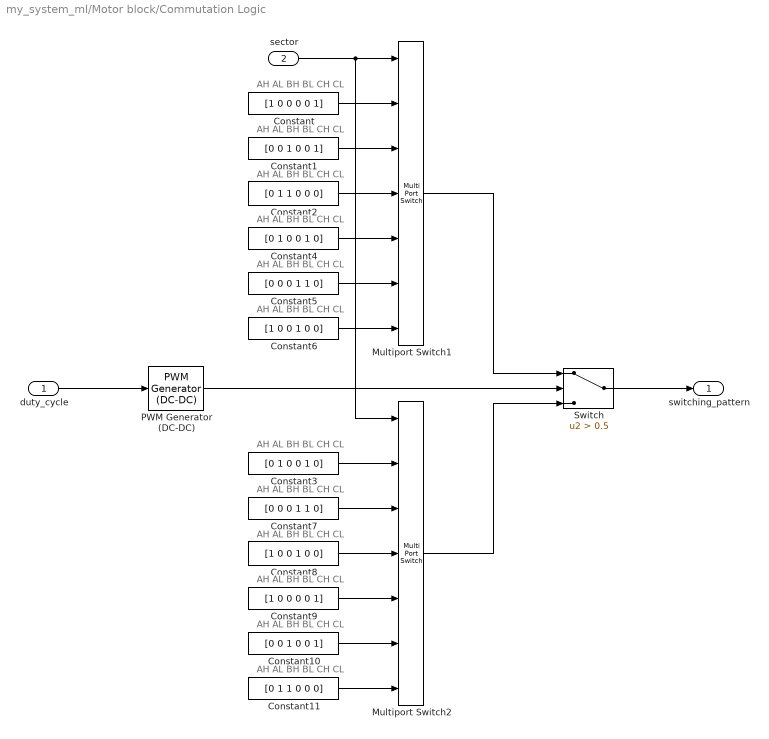
== system my_system_ml/Motor block/Commutation Logic ==
  note: AH AL BH BL CH CL
  note: AH AL BH BL CH CL
  note: AH AL BH BL CH CL
  note: AH AL BH BL CH CL
  note: AH AL BH BL CH CL
  note: AH AL BH BL CH CL
  note: AH AL BH BL CH CL
  note: AH AL BH BL CH CL
  note: AH AL BH BL CH CL
  note: AH AL BH BL CH CL
  note: AH AL BH BL CH CL
  note: AH AL BH BL CH CL
  duty_cycle : Inport
  sector : Inport  Port=2
  Constant : Constant  Value=[1 0 0 0 0 1]
  Constant1 : Constant  Value=[0 0 1 0 0 1]
  Constant10 : Constant  Value=[0 0 1 0 0 1]
  Constant11 : Constant  Value=[0 1 1 0 0 0]
  Constant2 : Constant  Value=[0 1 1 0 0 0]
  Constant3 : Constant  Value=[0 1 0 0 1 0]
  Constant4 : Constant  Value=[0 1 0 0 1 0]
  Constant5 : Constant  Value=[0 0 0 1 1 0]
  Constant6 : Constant  Value=[1 0 0 1 0 0]
  Constant7 : Constant  Value=[0 0 0 1 1 0]
  Constant8 : Constant  Value=[1 0 0 1 0 0]
  Constant9 : Constant  Value=[1 0 0 0 0 1]
  Multiport Switch1 : MultiPortSwitch  Inputs=6  SaturateOnIntegerOverflow=off  InputSameDT=off
  Multiport Switch2 : MultiPortSwitch  Inputs=6  SaturateOnIntegerOverflow=off  InputSameDT=off
  PWM Generator (DC-DC) : spsPWMGeneratorDCDCLib/PWM Generator (DC-DC)  Fsw=1000  Ts=Ts_motor
  Switch : Switch  Criteria=u2 > Threshold  Threshold=0.5  SaturateOnIntegerOverflow=off  InputSameDT=off
  "  switching_pattern" : Outport  VectorParamsAs1DForOutWhenUnconnected=off
  wires:
  duty_cycle/1 -> PWM Generator (DC-DC)/1
  PWM Generator (DC-DC)/1 -> Switch/2
  Multiport Switch2/1 -> Switch/3
  Constant7/1 -> Multiport Switch2/3
  Constant6/1 -> Multiport Switch1/7
  Constant2/1 -> Multiport Switch1/4
  Constant/1 -> Multiport Switch1/2
  Constant9/1 -> Multiport Switch2/5
  sector/1 -> Multiport Switch2/1, Multiport Switch1/1
  Constant11/1 -> Multiport Switch2/7
  Constant10/1 -> Multiport Switch2/6
  Constant3/1 -> Multiport Switch2/2
  Multiport Switch1/1 -> Switch/1
  Constant8/1 -> Multiport Switch2/4
  Switch/1 -> "  switching_pattern"/1
  Constant4/1 -> Multiport Switch1/5
  Constant1/1 -> Multiport Switch1/3
  Constant5/1 -> Multiport Switch1/6

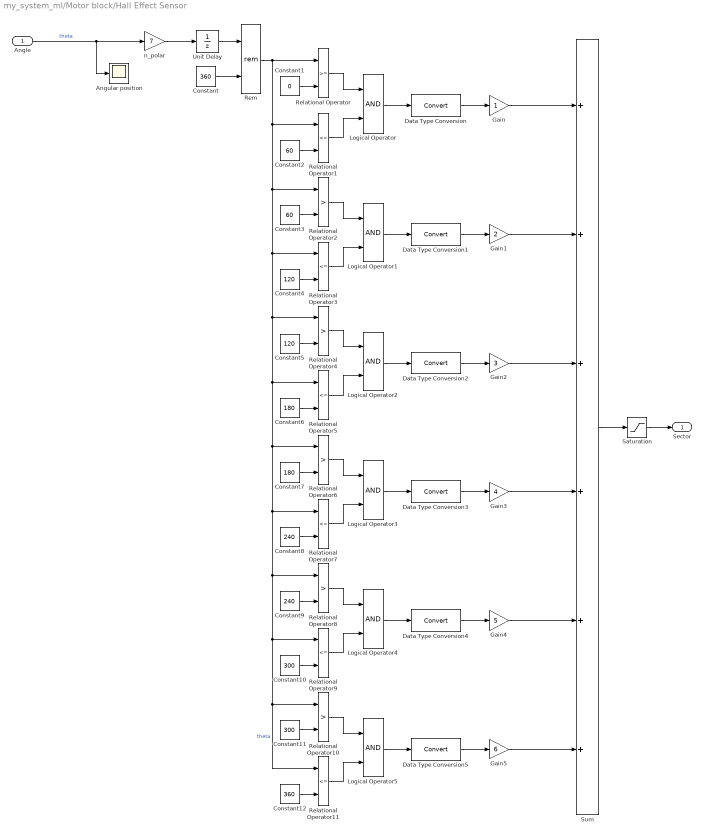
== system my_system_ml/Motor block/Hall Effect Sensor ==
  Angle : Inport
  Angular position : Scope
  Constant : Constant  Value=360
  Constant1 : Constant  Value=0
  Constant10 : Constant  Value=300
  Constant11 : Constant  Value=300
  Constant12 : Constant  Value=360
  Constant2 : Constant  Value=60
  Constant3 : Constant  Value=60
  Constant4 : Constant  Value=120
  Constant5 : Constant  Value=120
  Constant6 : Constant  Value=180
  Constant7 : Constant  Value=180
  Constant8 : Constant  Value=240
  Constant9 : Constant  Value=240
  Data Type Conversion{,1..5} (6 alike) : DataTypeConversion  SaturateOnIntegerOverflow=off  RndMeth=Floor
  Gain : Gain
  Gain1 : Gain  Gain=2
  Gain2 : Gain  Gain=3
  Gain3 : Gain  Gain=4
  Gain4 : Gain  Gain=5
  Gain5 : Gain  Gain=6
  Logical Operator{,1..5} (6 alike) : Logic  AllPortsSameDT=off  OutDataTypeStr=boolean
  Relational Operator : RelationalOperator  OutDataTypeStr=boolean  RndMeth=Simplest  InputSameDT=off
  Relational Operator{1,3,5,7,9,11} (6 alike) : RelationalOperator  Operator=<=  OutDataTypeStr=boolean  RndMeth=Simplest  InputSameDT=off
  Relational Operator{2,4,6,8,10} (5 alike) : RelationalOperator  Operator=>  OutDataTypeStr=boolean  RndMeth=Simplest  InputSameDT=off
  Rem : Math  Operator=rem
  Saturation : Saturate  UpperLimit=6  LowerLimit=1
  Sum : Sum  Inputs=++++++
  Unit Delay : UnitDelay  SampleTime=-1  HasFrameUpgradeWarning=on
  n_polar : Gain  Gain=7
  Sector : Outport
  wires:
  Constant12/1 -> Relational Operator11/2
  Logical Operator2/1 -> Data Type Conversion2/1
  Constant7/1 -> Relational Operator6/2
  Gain4/1 -> Sum/5
  Gain/1 -> Sum/1
  Relational Operator10/1 -> Logical Operator5/1
  Relational Operator8/1 -> Logical Operator4/1
  Constant5/1 -> Relational Operator4/2
  Rem/1 -> Relational Operator11/1, Relational Operator10/1, Relational Operator9/1, Relational Operator8/1, Relational Operator7/1, Relational Operator6/1, Relational Operator5/1, Relational Operator4/1, Relational Operator3/1, Relational Operator2/1, Relational Operator1/1, Relational Operator/1  "theta"
  Constant10/1 -> Relational Operator9/2
  Relational Operator9/1 -> Logical Operator4/2
  Unit Delay/1 -> Rem/1
  Logical Operator3/1 -> Data Type Conversion3/1
  Logical Operator/1 -> Data Type Conversion/1
  Constant9/1 -> Relational Operator8/2
  Data Type Conversion4/1 -> Gain4/1
  Logical Operator4/1 -> Data Type Conversion4/1
  Relational Operator/1 -> Logical Operator/1
  Relational Operator3/1 -> Logical Operator1/2
  Angle/1 -> n_polar/1, Angular position/1  "theta"
  Gain3/1 -> Sum/4
  Gain1/1 -> Sum/2
  Relational Operator2/1 -> Logical Operator1/1
  Logical Operator5/1 -> Data Type Conversion5/1
  Constant4/1 -> Relational Operator3/2
  Relational Operator11/1 -> Logical Operator5/2
  Constant8/1 -> Relational Operator7/2
  n_polar/1 -> Unit Delay/1
  Constant3/1 -> Relational Operator2/2
  Logical Operator1/1 -> Data Type Conversion1/1
  Data Type Conversion1/1 -> Gain1/1
  Constant1/1 -> Relational Operator/2
  Relational Operator4/1 -> Logical Operator2/1
  Constant6/1 -> Relational Operator5/2
  Relational Operator5/1 -> Logical Operator2/2
  Relational Operator7/1 -> Logical Operator3/2
  Data Type Conversion2/1 -> Gain2/1
  Data Type Conversion3/1 -> Gain3/1
  Relational Operator6/1 -> Logical Operator3/1
  Data Type Conversion5/1 -> Gain5/1
  Gain2/1 -> Sum/3
  Data Type Conversion/1 -> Gain/1
  Relational Operator1/1 -> Logical Operator/2
  Constant/1 -> Rem/2
  Gain5/1 -> Sum/6
  Constant2/1 -> Relational Operator1/2
  Constant11/1 -> Relational Operator10/2
  Sum/1 -> Saturation/1
  Saturation/1 -> Sector/1
